simulink model "Method_2_Slip_Ratio_Based"  (R2020b)
settings: Solver=VariableStepAuto  StartTime=0.0  StopTime=100  RelTol=1e-3
values from neighbouring files (symbols this model uses):
  GR = 5    [Model_Data.mat]
  m = 220    [Model_Data.mat]
  r = 0.3059    [Model_Data.mat]
  s2_5_rps = [0 104.6666667 209.3333333 314 418.6666667 523.3333333 628]    [Model_Data.mat]
  s2_5_trq = [70 65 60 50 40 33 27]    [Model_Data.mat]
undefined symbols (not defined in the file or in its folder): h, km, s, sigbuilder_block
libraries: autolibshared x4, aerolibconvert2 x2, autolibmappedmotor x1, simulink x1
(part 3 of 3)

== matlab function Method_2_Slip_Ratio_Based/Traction Controller ==
  data: Slip_Ratio input; acc_out output; Driver_Command input
function acc_out  = fcn(Slip_Ratio,Driver_Command)

if (Slip_Ratio<0.2)
    acc_out = Driver_Command;
end

if (Slip_Ratio>0.2 && Slip_Ratio<2)
    acc_out = 0.8*Driver_Command;
end

if (Slip_Ratio>2 && Slip_Ratio<5)
    acc_out = 0.6*Driver_Command;
end

if (Slip_Ratio>5)
    acc_out = 0.4*Driver_Command;

else
    acc_out = Driver_Command;
end

            
 end
